simulink library "vpc_new"  (Simulink 8.1)
settings: Solver=ode1  StartTime=0.0  StopTime=Inf  FixedStep=0.001  RelTol=1e-3
PostLoadFcn:
  | , if any(exist('dsrtsu_mdlpostloadfcn', 'file') == [2, 3, 6]), try dsrtsu_mdlpostloadfcn('Execute', bdroot); catch fprintf('Error in PostLoadFcn (dsrtsu_mdlpostloadfcn) for model "%s":\n %s\n', bdroot, lasterr); end, end,
undefined symbols (not defined in the file or in its folder): KIFO_HostVehicleWidth_m, KIFO_PedestrianWidth_m, KIFO_VRUPotentiallityLimit_perc
libraries: ipc x2, poc_new x1
settings Model: DSRTSU_INTERNAL_RTI_VER=450  DSRTSU_INTERNAL_RTI_TYPE=rti1401  RTICANMMDATA=struct('GeneralSetupData',struct('modelroot','D:\PROJECTS\HAITEC\TAIWAN_HAITEC_SVN\trunk\AdasDragon\software\sw_development\arch\app\ifo','generalsettings',struct('filesettings',struct('destfolder',struct('Name','RTICANMM_FILES','Check',1),'buildfolder',struct('Name','.','Check',1),'AbsDestfolder',struct('Name','D:\PROJECTS\HAITEC\TAIWAN_HAITEC_SVN\trunk\AdasDragon\software\sw_development\arch\app\ifo\RTICANMM_FILES'),'AbsBuildfolder',struct('Name','D:\PROJECTS\HAITEC\TAIWAN_HAITEC_SVN\trunk\AdasDragon\software\sw_development\arch\app\ifo'))),'options',struct('addpaths',1,'rmpaths',1,'addtrcexclusion',logical(1),'cannavigator',struct('checkmonitoring',0),'show_usrtrc',0,'use_usrtrc',0),'advanced',struct('options',[1 1 1 1 1 1 1 1 1 1 1 1 1 1 1 1 1 1 1 1 1 1 1 1 1 1 1 1 1 1 1 1 1 1 1 1 1 1 1 1 1 1 1 1 1 1 1 1 1 1 1 1 1 1 1 1 1 1 1 1 1 1 1 1 1 1 1 1 1 1 1 1 1 1 1 1 1 1 1 1 1 1 1 1 1 1 1 1 1 1 1 1 1 1 1 1 1 1 1 1]),'MPSetup',{{}},'modelname','vpc_new','block','vpc_new'))  DSRTSU_INTERNAL_RTIFPGA=40  Creator=tescamilla  LastModifiedBy=tescamilla

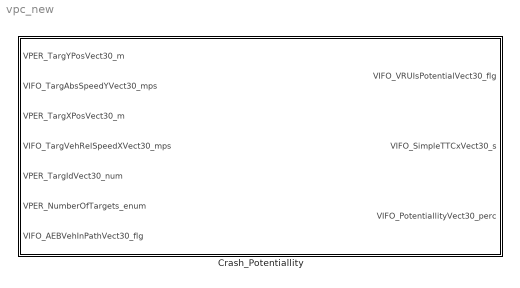
== system vpc_new ==
  Crash_Potentiallity : Subsystem

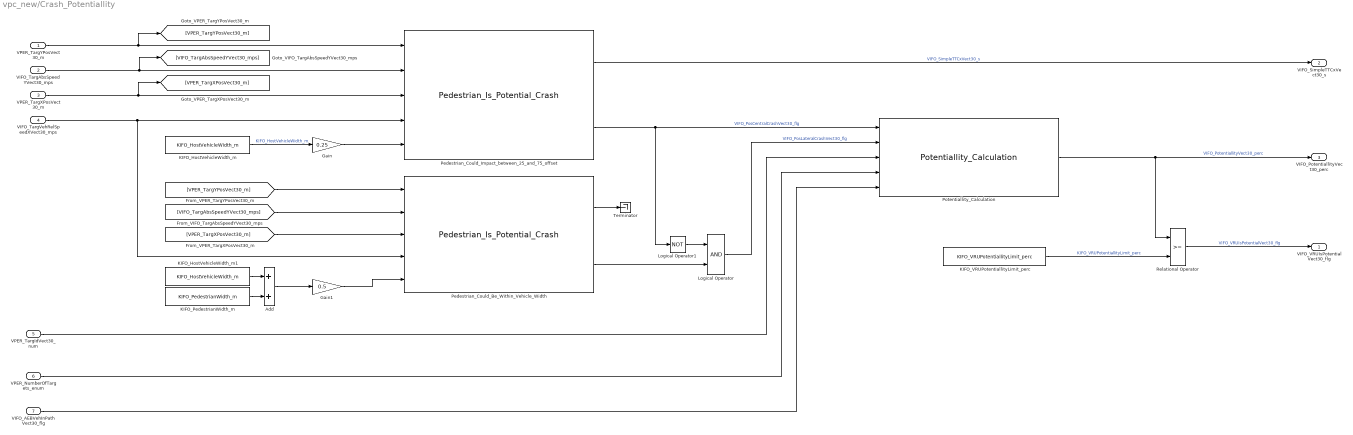
== system vpc_new/Crash_Potentiallity ==
  VPER_TargYPosVect30_m : Inport
  VIFO_TargAbsSpeedYVect30_mps : Inport  Port=2
  VPER_TargXPosVect30_m : Inport  Port=3
  VIFO_TargVehRelSpeedXVect30_mps : Inport  Port=4
  VPER_TargIdVect30_num : Inport  Port=5
  VPER_NumberOfTargets_enum : Inport  Port=6
  VIFO_AEBVehInPathVect30_flg : Inport  Port=7
  Add : Sum
  Gain : Gain  Gain=0.25
  Gain1 : Gain  Gain=0.5
  KIFO_HostVehicleWidth_m : Constant  Value=KIFO_HostVehicleWidth_m
  KIFO_HostVehicleWidth_m1 : Constant  Value=KIFO_HostVehicleWidth_m
  KIFO_PedestrianWidth_m : Constant  Value=KIFO_PedestrianWidth_m
  KIFO_VRUPotentiallityLimit_perc : Constant  Value=KIFO_VRUPotentiallityLimit_perc
  Logical Operator : Logic  AllPortsSameDT=off  OutDataTypeStr=boolean
  Logical Operator1 : Logic  Operator=NOT  AllPortsSameDT=off  OutDataTypeStr=boolean
  Pedestrian_Could_Be_Within_Vehicle_Width : ipc/Pedestrian_Is_Potential_Crash
  Pedestrian_Could_Impact_between_25_and_75_offset : ipc/Pedestrian_Is_Potential_Crash
  Potentiallity_Calculation : poc_new/Potentiallity_Calculation
  Relational Operator : RelationalOperator  OutDataTypeStr=boolean
  Terminator : Terminator
  VIFO_VRUIsPotentialVect30_flg : Outport
  VIFO_SimpleTTCxVect30_s : Outport  Port=2
  VIFO_PotentiallityVect30_perc : Outport  Port=3
  wires:
  VIFO_AEBVehInPathVect30_flg/1 -> Potentiallity_Calculation/5
  Add/1 -> Gain1/1
  KIFO_PedestrianWidth_m/1 -> Add/2
  KIFO_HostVehicleWidth_m1/1 -> Add/1
  VPER_NumberOfTargets_enum/1 -> Potentiallity_Calculation/4
  VPER_TargIdVect30_num/1 -> Potentiallity_Calculation/3
  Pedestrian_Could_Be_Within_Vehicle_Width/1 -> Terminator/1
  Pedestrian_Could_Impact_between_25_and_75_offset/1 -> VIFO_SimpleTTCxVect30_s/1  "VIFO_SimpleTTCxVect30_s"
  Relational Operator/1 -> VIFO_VRUIsPotentialVect30_flg/1  "VIFO_VRUIsPotentialVect30_flg"
  KIFO_VRUPotentiallityLimit_perc/1 -> Relational Operator/2  "KIFO_VRUPotentiallityLimit_perc"
  Potentiallity_Calculation/1 -> VIFO_PotentiallityVect30_perc/1, Relational Operator/1  "VIFO_PotentiallityVect30_perc"
  Logical Operator/1 -> Potentiallity_Calculation/2  "VIFO_PosLateralCrashVect30_flg"
  [VPER_TargYPosVect30_m] -> Pedestrian_Could_Be_Within_Vehicle_Width/1
  [VPER_TargXPosVect30_m] -> Pedestrian_Could_Be_Within_Vehicle_Width/3
  [VIFO_TargAbsSpeedYVect30_mps] -> Pedestrian_Could_Be_Within_Vehicle_Width/2
  Gain1/1 -> Pedestrian_Could_Be_Within_Vehicle_Width/5
  Gain/1 -> Pedestrian_Could_Impact_between_25_and_75_offset/5
  Pedestrian_Could_Impact_between_25_and_75_offset/2 -> Potentiallity_Calculation/1, Logical Operator1/1  "VIFO_PosCentralCrashVect30_flg"
  VIFO_TargAbsSpeedYVect30_mps/1 -> Pedestrian_Could_Impact_between_25_and_75_offset/2, [VIFO_TargAbsSpeedYVect30_mps]
  VPER_TargYPosVect30_m/1 -> Pedestrian_Could_Impact_between_25_and_75_offset/1, [VPER_TargYPosVect30_m]
  VIFO_TargVehRelSpeedXVect30_mps/1 -> Pedestrian_Could_Impact_between_25_and_75_offset/4, Pedestrian_Could_Be_Within_Vehicle_Width/4
  VPER_TargXPosVect30_m/1 -> Pedestrian_Could_Impact_between_25_and_75_offset/3, [VPER_TargXPosVect30_m]
  KIFO_HostVehicleWidth_m/1 -> Gain/1  "KIFO_HostVehicleWidth_m"
  Pedestrian_Could_Be_Within_Vehicle_Width/2 -> Logical Operator/2
  Logical Operator1/1 -> Logical Operator/1
